simulink model "RM3"  (R2020b)
settings: Solver=ode4  StartTime=0  StopTime=400  FixedStep=0.1  RelTol=1e-3  EnableMultiTasking=on
undefined symbols (not defined in the file or in its folder): body, constraint, geometry, hydroData, pto
libraries: WECSim_Lib_Body x2, WECSim_Lib_Frames x1, WECSim_Lib_Constraints x1, WECSim_Lib_PTOs x1
settings Model: Creator=mlawson  LastModifiedBy=kmruehl
settings SolverCC: AlgebraicLoopSolver=LineSearch
settings DataIOCC: SaveFormat=Array  SaveOutput=off  SaveTime=off  ReturnWorkspaceOutputs=off
settings OptimizationCC: LifeSpan=inf
settings DebuggingCC: UnderspecifiedInitializationDetection=Classic  MergeDetectMultiDrivingBlocksExec=none  SolverPrmCheckMsg=warning  AllowSymbolicDim=off  StateNameClashWarn=warning  SFUnexpectedBacktrackingDiag=warning  SFNoUnconditionalDefaultTransitionDiag=warning  SFExecutionAtInitializationDiag=none  ArithmeticOperatorsInVariantConditions=warning
settings HardwareCC: ProdBitPerPointer=32  ProdBitPerSizeT=32  ProdBitPerPtrDiffT=32  ProdLargestAtomicFloat=None  ProdIntDivRoundTo=Undefined  ProdEndianess=Unspecified  ProdWordSize=32  ProdHWDeviceType=32-bit Generic
settings ModelReferenceCC: PropagateSignalLabelsOutOfModel=off
settings SFSimCC: SimUseLocalCustomCode=off  CustomCodeUndefinedFunction=UseInterfaceOnly
settings RTWCC: RTWUseLocalCustomCode=off
settings CodeAppCC: StateflowObjectComments=on
settings GRTTargetCC: TargetLangStandard=C89/C90 (ANSI)
settings ConfigComp: CovMetricSettings=dw  CovSaveCumulativeToWorkspaceVar=on  CovSaveSingleToWorkspaceVar=on  CovExternalEMLEnable=off  CovSFcnEnable=off
settings SimscapeCC: SimscapeNormalizeSystem=off
settings ConfigurationSet: Description=SimMechanics 2G
settings ExplorerConfigSet: InternalSimMechanicsExplorerSettings="<ExplorerConfiguration><canonicalview>default</canonicalview><TilePanel><TileInfo><Tiles Columns=\"1\" Count=\"1\" Rows=\"1\"><Column Left=\"2\" Weight=\"1\"/><Column Left=\"1335\"/><Row Top=\"2\" Weight=\"1\"/><Row Top=\"911\"/><Tile Height=\"1\" Width=\"1\" X=\"0\" Y=\"0\"/></Tiles></TileInfo><SceneInfo><SceneViewer><BGColor><R>0.60000002384185791</R><G>0.60000002384185791</G><B>0.60000002384185791</B></BGColor><Camera><Position><X>365.37645888990272</X><Y>-369.82486814446582</Y><Z>359.64809521743916</Z></Position><Center><X>-6.7351450971904585</X><Y>2.2867358426280204</Y><Z>-12.463508769654169</Z></Center><Up><X>-0.40824829046386307</X><Y>0.40824829046386307</Y><Z>0.81649658092772615</Z></Up><Left>-57.820127362122818</Left><Right>57.820127362122818</Right><Bottom>-38.308817187253304</Bottom><Top>38.308817187253304</Top></Camera></SceneViewer></SceneInfo></TilePanel></ExplorerConfiguration>"

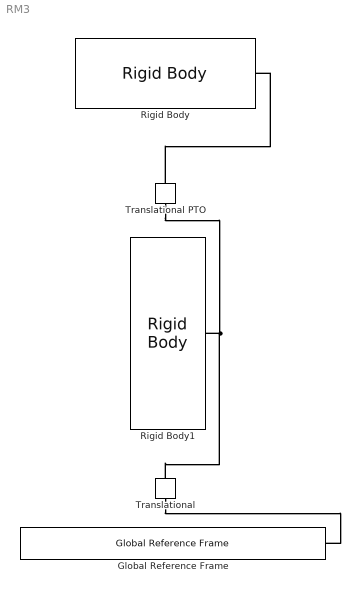
== system RM3 ==
  Global Reference Frame : WECSim_Lib_Frames/Global Reference Frame  waves=waves  simu=simu  ParamInput=Custom Parameters  InputFile=wecSimInputFile.m  mode=normal  explorer=off  solver=ode4  startTime=0  rampTime=100  endTime=400  dt=0.1  CITime=60  ssCalc=0  morisonElement=0  WaveClass=regular  H=2.5  T=8  etaDataFile=NOT DEFINED  spectrumDataFile=NOT DEFINED  waveDir=0  waveSpread=1  spectrumType=NOT DEFINED  freqDisc=EqualEnergy  phaseSeed=0
  Rigid Body : WECSim_Lib_Body/Rigid Body  body=body(1)  h5File=hydroData/*.h5  geometryFile=geometry/*.stl  mass=0  momOfInertia=0 0 0  nhBody=0  cg=0 0 0  cb=0 0 0  dof=6  dispVol=0  initLinDisp=0 0 0  initAngularDispAxis=0 1 0  initAngularDispAngle=0  cd=0 0 0  ca=0 0 0  characteristicArea=0 0 0  VME=0  rgME=0 0 0  z=0 0 1
      settings: AttributesFormatString=%<body>
  Rigid Body1 : WECSim_Lib_Body/Rigid Body  body=body(2)  h5File=hydroData/*.h5  geometryFile=geometry/*.stl  mass=0  momOfInertia=0 0 0  nhBody=0  cg=0 0 0  cb=0 0 0  dof=6  dispVol=0  initLinDisp=0 0 0  initAngularDispAxis=0 1 0  initAngularDispAngle=0  cd=0 0 0  ca=0 0 0  characteristicArea=0 0 0  VME=0  rgME=0 0 0  z=0 0 1
      settings: AttributesFormatString=%<body>
  Translational : WECSim_Lib_Constraints/Translational  constraint=constraint(1)  loc="0  0  0"  initLinDisp=0 0 0  y=0 1 0  z=0 0 1  upperLimitSpecify=off  upperLimitBound=0  upperLimitTransitionRegionWidth=0  upperLimitStiffness=0  upperLimitDamping=0  lowerLimitSpecify=off  lowerLimitBound=0  lowerLimitTransitionRegionWidth=0  lowerLimitStiffness=0  lowerLimitDamping=0
      settings: AttributesFormatString=%<constraint>
  Translational PTO : WECSim_Lib_PTOs/Translational PTO  pto=pto(1)  loc="0  0  0"  k=0  c=0  equilibriumPosition=0  pretension=0  initLinDisp=0 0 0  y=0 1 0  z=0 0 1  upperLimitSpecify=off  upperLimitBound=0  upperLimitTransitionRegionWidth=0  upperLimitStiffness=0  upperLimitDamping=0  lowerLimitSpecify=off  lowerLimitBound=0  lowerLimitTransitionRegionWidth=0  lowerLimitStiffness=0  lowerLimitDamping=0
      settings: AttributesFormatString=%<pto>
  connections:
  Translational/LConn1 -- Global Reference Frame/RConn1
  Rigid Body1/RConn1 -- Translational/RConn1 -- Translational PTO/RConn1
  Translational PTO/LConn1 -- Rigid Body/RConn1
